simulink model "test_com_SensorFusion_SF_D4_ukf"  (R2019b)
settings: Solver=FixedStepDiscrete  StartTime=0  StopTime=stop  FixedStep=0.001  RelTol=1e-3
undefined symbols (not defined in the file or in its folder): breakpoints_camber_posZ, breakpoints_camber_RollAngle, BxTM, ByTM, camber_posZ_rear, camber_RollAngle_front, camber_RollAngle_rear, CxTM, CyTM, enable_kalman_standing, enable_simpleTireLoad_pGL, enable_v2o_direct, g, gamma_stat_front, gamma_stat_rear, gearbox_ratio, l_F, l_R, m_sprung, m_unsprung_quarter, mag_calib_front_center, mag_calib_front_compmatrix, mag_calib_rear_center, mag_calib_rear_compmatrix, should_be_in_theSensorFusion, switch_lat_accel_tireloadestimE8, switch_rocker_direction_FL, switch_rocker_direction_FR, switch_rocker_direction_RL, switch_rocker_direction_RR, switch_VelYcalculation_pSF, testStart_VelX_pSF, testVelY_pSF, tire_r_dyn, track_angle_front, track_width_front, track_width_rear, v2o_x, wheel_kinematics_breakpoints, wheel_kinematics_FL_data, wheel_kinematics_FR_data, wheelbase, x9DFrontX, x9DFrontY, x9DRearX, x9DRearY
libraries: SignalProcessingSensorFusionLib x30, simulink x9
(part 8 of 9)

== matlab function test_com_SensorFusion_SF_D4_ukf/Subsystem14/SensorFusion_D4/SF_LaKl_ukf ==
  data: x9DFront input Bus: control_9D; VehicleState output Bus: control_VehicleState; used_bias output Bus: control_bias_kalman_SiDe; used_measurements output Bus: control_used_measurements_SiDe; x9DRear input Bus: control_9D; v2o input Bus: control_Velocity; WheelSpeeds input; WheelSpeeds_Sq input; RockerAngle input; RockerAngle_Sq input; dt input; SteeringAngle input; bias_measurement_running output; kalman_running output; TireLoad output; TireSlipAngle output; TireSlipLong output; tire_r_dyn parameter; Rolling output; Pitching output; spring_stiff_roll_rear parameter; spring_stiff_heave_rear parameter; tire_cornering_stiffness parameter; wheel_inertia parameter; m_sprung parameter; m_unsprung_quarter parameter; damp_coef_heave_front_push parameter; damp_coef_heave_front_pull parameter; damp_coef_heave_rear_push parameter; damp_coef_roll_front_pull parameter; track_width_front parameter; track_width_rear parameter; spring_stiff_heave_front parameter; motion_ratio_heave_front parameter; motion_ratio_heave_rear parameter; wheelbase parameter; spring_stiff_roll_front parameter; motion_ratio_roll_front parameter; motion_ratio_roll_rear parameter; l_F parameter; l_R parameter; WheelTorque input; WheelAngle_FL input; WheelAngle_FR input; damp_coef_roll_front_push parameter; damp_coef_roll_rear_pull parameter; damp_coef_roll_rear_push parameter; damp_coef_heave_rear_pull parameter; Fx_tf_long input; Fy_tf_lat input; vehicle_inertia_yaw parameter; Fx_tf_long output; C_tl output; D_tl output; VelZ_eval output; PosZ output; TireLoad_z input; J_Sxx input; J_Syy input; x9DFrontX input; v2o_x input; chi output
function [VehicleState,used_bias,used_measurements,bias_measurement_running,kalman_running ,TireLoad, TireSlipAngle, TireSlipLong ,Rolling, Pitching, Fx_tf_long, C_tl,   D_tl, VelZ_eval, PosZ, chi]  = fcn(x9DFront, x9DRear, v2o, WheelSpeeds, WheelSpeeds_Sq, RockerAngle, RockerAngle_Sq, dt, SteeringAngle, tire_r_dyn,spring_stiff_roll_rear, spring_stiff_heave_rear, tire_cornering_stiffness, wheel_inertia, m_sprung, m_unsprung_quarter, damp_coef_heave_front_push, damp_coef_heave_front_pull, damp_coef_heave_rear_push, damp_coef_roll_front_pull, track_width_front, track_width_rear, spring_stiff_heave_front, motion_ratio_heave_front, motion_ratio_heave_rear, wheelbase, spring_stiff_roll_front, motion_ratio_roll_front, motion_ratio_roll_rear, l_F, l_R, WheelTorque, WheelAngle_FL, WheelAngle_FR, damp_coef_roll_front_push, damp_coef_roll_rear_pull, damp_coef_roll_rear_push, damp_coef_heave_rear_pull,Fx_tf_long, Fy_tf_lat, vehicle_inertia_yaw, TireLoad_z, J_Sxx, J_Syy, x9DFrontX, v2o_x)
%% SAE is the used KOS, global not local on the car -> trafo of measurements in global KOS necessary, but vel is local on the car?
persistent state P

persistent standstill_counter
persistent bias_measurements 
persistent P_bias

persistent YawAngle_Front_old YawAngle_Rear_old v2o_VelX_old RollAngle_Front_old PitchAngle_Front_old
persistent TireLoad_old chi_velocity velocity_old


num_states= 12;
num_measurements=7;


% state   =   (1) PosX
%             (2) PosY
%             (3) PosZ
%             (4) VelX
%             (5) VelY
%             (6) VelZ
%             (7) YawAngle
%             (8) RollAngle
%             (9) PitchAngle
%             (10) YawRate

     

% Actually used measurements:
%               (1) VelX
%               (2) VelY
%               (3) YawRate
%               (4) RollRate
%               (5) PitchRate



if isempty(P)
    
    P_bias=single(eye(num_measurements));%*0.01;
    standstill_counter=0;
    bias_measurements=single(zeros(num_measurements,1));
    

    state = single(zeros(num_states,1));
    P = single(eye(num_states, num_states)*10);
    
    YawAngle_Front_old=single(0);
    YawAngle_Rear_old=single(0);
    v2o_VelX_old=single(0);
    TireLoad_old= single([m_unsprung_quarter+0.5*m_sprung*l_R/wheelbase; ...
        m_unsprung_quarter + 0.5*m_sprung*l_R/wheelbase; ...
        m_unsprung_quarter + 0.5*m_sprung*l_F/wheelbase; ...
        m_unsprung_quarter + 0.5*m_sprung*l_F/wheelbase]);
    Fx_tf_long(1:4)=0;
    Fy_tf_lat(1:4)=0;
    chi_velocity = 0;
    velocity_old = [0;0];
end




%% Readability

PosX=       state(1);
PosY=       state(2);
PosZ=       state(3);
VelX=       state(4);
VelY=       state(5);
VelZ=       state(6);
RollAngle = state(7);
PitchAngle= state(8);
YawAngle=   state(9);
RollRate = state(10);
PitchRate = state(11);
YawRate =   state(12);

AccX_measurement = x9DFront.AccX;
AccY_measurement = x9DFront.AccY;
AccZ_measurement = x9DFront.AccZ;
YawRate_measurement = x9DFront.YawRate*1.167;%*0.8569;%; % the E9 Sensor had a wrong YawRate %*0.8569;%
RollRate_measurement = x9DFront.RollRate;
PitchRate_measurement = x9DFront.PitchRate;

chi = single(chi_velocity);

if isempty(YawAngle_Front_old)
    YawAngle_Front_old = single(0);
end
% 
if isempty(RollAngle_Front_old)
    RollAngle_Front_old = single(0);
end

if isempty(PitchAngle_Front_old)
    PitchAngle_Front_old = single(0);
end
YawAngle_measurement = single(0); %YawAngle_Front_old; %; 
RollAngle_measurement =  single(0);%RollAngle_Front_old; %
PitchAngle_measurement = single(0);% PitchAngle_Front_old;%
PosZ_measurement = single(0);
VelZ_measurement = single(0);

    measurements= [
        PosZ_measurement
v2o.VelX              % (1)  v2o Sensor  x velocity
v2o.VelY              % (2)  v2o Sensor  y velocity
VelZ_measurement
% RollAngle_measurement
% PitchAngle_measurement
RollRate_measurement
PitchRate_measurement
YawRate_measurement
];
% unused Pfusch-measurements (either integrating or giving zero dynamics)
% YawAngle_measurement
% RollAngle_measurement
% PitchAngle_measurement
% PosZ_measurement


measurements_Sq= [
    0
v2o.VelX_Sq            % (1)   v2o Sensor x velocity         Signal Quality
v2o.VelY_Sq            % (2)   v2o Sensor y velocity         Signal Quality
0
0
0
0];



%Correction of the sensor inputs with the estimated biases
% nb == no bias
measurements_nb=    measurements-bias_measurements;
PosZ_nb =           measurements_nb(1);
v2o_VelX_nb=        measurements_nb(2);
v2o_VelY_nb=        measurements_nb(3);
VelZ_nb=            measurements_nb(4);
% AccX_nb =           measurements_nb(5);
% AccY_nb =           measurements_nb(6);
% AccZ_nb =           measurements_nb(7);
% RollAngle_nb =      measurements_nb(8);
% PitchAngle_nb =     measurements_nb(9);
%YawAngle_nb =       measurements_nb(10);
RollRate_nb =       measurements_nb(5);
PitchRate_nb =      measurements_nb(6);
YawRate_nb =        measurements_nb(7);                

Q=diag([0.00001   %(1) PosX 01E-8
        0.0001   %(2) PosY 01E-8
        0.001    %(3) PosZ 1E-6
        0.001    %(4) VelX 0.001
        0.001     %(5) VelY 0.001
        1    %(6) VelZ 0,1 
        0.0001    %(10) RollAngle 0.001
        0.0001   % (11)  PitchAngle 0.0001
        0.00001    %(12) YawAngle 0.001
        0.00001    %(13)RollRate
        0.00001      %(14) PitchRate
        0.00001]);   %(15) YawRate 

%Measurement noise Covariance matrix
    
R=diag([0.01  %(1) PosZ
        0.01   % (1) VelX 1E-3
        0.01   % (2) VelY 1E-3
        1    % (3) VelZ 
        0.001    % (7) RollRate
        0.001   % (8) PitchRate
        0.001 ]);   % (7) YawRate
%         0.001    % (8) PitchRate 
%         0.0001 % (9) YawRate 
%         
     
avgWheelSpeed=mean(abs(WheelSpeeds));


if (avgWheelSpeed < 0.02 )
        vehicle_is_driving=false;
        standstill_counter=standstill_counter+1;
else
        vehicle_is_driving=true;
        standstill_counter=0;
end

bias_measurement_running=false;
kalman_running=false;

%vehicle_is_driving = true;

RollAngle = state(8);
PitchAngle = state(9);

%Verwendete Messung für v2o VelX
use_v2o_VelX=0;
v2o_VelX_used_measurement=single(0);
if (v2o.VelX_Sq<4) && (v2o.VelY_Sq<4) && abs(v2o_VelX_nb-v2o_VelX_old) < 2
    
    v2o_VelX_used_measurement=v2o_VelX_nb;

    use_v2o_VelX=1;

end

if(v2o_VelX_old~=v2o_VelX_nb)
    v2o_VelX_old=v2o_VelX_nb;
end

% 0.221 = r_dyn vom Reifen : v = r*omega
% Chi square test to validate velocity measurement and estimation
if chi_velocity>4
    v2o_VelX_nb = single((WheelSpeeds(3)+WheelSpeeds(4)+cosd(SteeringAngle)*(WheelSpeeds(1)+WheelSpeeds(2)))*0.221/(4));
    v2o_VelY_nb = single(sind(SteeringAngle)*(WheelSpeeds(1)+WheelSpeeds(2))*0.221);
end


% measurement vector
zmeas  = [PosZ_nb;...
    v2o_VelX_nb;...
    v2o_VelY_nb;...
    VelZ_nb;...
    RollRate_nb;...
    PitchRate_nb;...
    YawRate_nb];

% calculate TF_Fx_front and TF_Fy_rear and TF_Fy_front

TF_Fx_F = Fx_tf_long(1)+Fx_tf_long(2);
TF_Fy_F = Fy_tf_lat(1)+Fy_tf_lat(2);
TF_Fy_R = Fy_tf_lat(3)+Fy_tf_lat(4);
TF_Fx_R = Fx_tf_long(3)+Fx_tf_long(4);

u = [WheelSpeeds(1);... % FL
    WheelSpeeds(2);...  % FR
    WheelSpeeds(3);...  % RL
    WheelSpeeds(4);...  % RR
    AccX_measurement;...
    AccY_measurement;...
    AccZ_measurement;...
    vehicle_inertia_yaw;...
    J_Sxx;...
    J_Syy;...
    TF_Fx_F;...
    TF_Fx_R;...
    TF_Fy_F;...
    TF_Fy_R;...
    TireLoad_z(1);...
    TireLoad_z(2);...
    TireLoad_z(3);...
    TireLoad_z(4);...
    SteeringAngle;...
    l_F;...
    l_R;...
    wheelbase;...
    track_width_front;...
    track_width_rear];

u_param = [x9DFrontX
    v2o_x];


%% Kalman-Filtering START
if (~vehicle_is_driving)
    

    if standstill_counter*dt>2 && standstill_counter*dt<10
    bias_measurement_running=true;    
    kill_matrix_bias=zeros(num_measurements,num_measurements);
        for i=1:num_measurements
            if measurements_Sq(i)<4
                kill_matrix_bias(i,i)=1;
            end
        end
        H_bias=kill_matrix_bias;
        R_bias=eye(num_measurements)*0.01;  % Sinnvolle Werte?
        I_bias=eye(num_measurements);
        
        Z_bias = kill_matrix_bias*measurements;
        w_bias = Z_bias-(H_bias*bias_measurements);
        K_bias = (P_bias*H_bias')/(H_bias*P_bias*H_bias.'+R_bias);  
        bias_measurements = bias_measurements+K_bias*w_bias;
        P_bias = (I_bias-K_bias*H_bias)*P_bias;
    end

    
    
    
    
else 
        
    kalman_running=true;
    fstate = @(x)f(x,u,dt);
    hmeas =@(x)h(x, u_param);



    % Unscented Kalman Filtering 
    [state,P,S,r1,r2]=ukf(fstate,state,P,hmeas,zmeas,Q,R);

    % try chi-square test for velocity
    r = r2(2:3)-r1(2:3);
    chi = r'*inv(S(2:3,2:3))*r;

    % if chi > bestimmter value -> von V2O auf Wheelspeeds als Signal umsteigen
    chi_velocity = double(chi);
end


% Plausibility check
if VelX<0
    VelX=single(0);
end

if ~vehicle_is_driving
    VelX=single(0); 
    VelY=single(0); 
    YawRate=single(0); 
end




VehicleState.PosX = PosX; % state(1);
VehicleState.PosY = PosY; % state(2);
VehicleState.VelX = VelX; % state(4);
VehicleState.VelY = VelY; % state(5);
VehicleState.YawAngle = YawAngle; % state(9);
VehicleState.YawRate = YawRate; % state(12);
VehicleState.YawAcc = single(0);
VehicleState.AccX = AccX_measurement;
VehicleState.AccY = AccY_measurement;
VehicleState.AccZ = AccZ_measurement;
VehicleState.isDriving = vehicle_is_driving;

Rolling = RollAngle;% state(7);
Pitching = PitchAngle; % state(8);
YawRate = YawRate; % state(12);

used_bias.VelX_bias=bias_measurements(1);
used_bias.VelY_bias=bias_measurements(2);
used_bias.YawAngle_9DFront_bias= single(0); %bias_measurements(3);
used_bias.YawRate_9DFront_bias=single(0); %bias_measurements(4);
used_bias.YawAngle_9DRear_bias=single(0);
used_bias.YawRate_9DRear_bias=single(0);
used_bias.wheelvelocity_FL_bias=single(0); %bias_measurements(5);
used_bias.wheelvelocity_FR_bias=single(0); %bias_measurements(6);
used_bias.wheelvelocity_RL_bias=single(0); %bias_measurements(7);
used_bias.wheelvelocity_RR_bias=single(0); %bias_measurements(8);


used_measurements.VelX_measurement=zmeas(1);
used_measurements.VelY_measurement=zmeas(2);
used_measurements.YawAngle_9DFront_measurement = single(0); %z(3);


used_measurements.YawRate_9DFront_measurement=zmeas(7); %z(4);
used_measurements.YawAngle_9DRear_measurement=single(0);
used_measurements.YawRate_9DRear_measurement=single(0);
used_measurements.wheelvelocity_FL_measurement=single(0); %z(5);
used_measurements.wheelvelocity_FR_measurement=single(0); %z(6);
used_measurements.wheelvelocity_RL_measurement=single(0); %z(7);
used_measurements.wheelvelocity_RR_measurement=single(0); %z(8);
YawAngle_Front_old = state(12);
RollAngle_Front_old = state(10);
PitchAngle_Front_old = state(11);
VelZ_eval = state(6);

%% Tire Load Estimation to improve Yaw Angle Estimation

% formula: tl= C_tl+D_tl;

% MonoShock Auswahl Druck/Zug-Stufe
if -PitchRate*l_F + PosZ > 0  %Vorne Druck
    damp_coef_heave_front = damp_coef_heave_front_push;
else                    %Vorne Zug
    damp_coef_heave_front = damp_coef_heave_front_pull;
end

if PitchRate*l_R + PosZ > 0  %Hinten Druck
    damp_coef_heave_rear = damp_coef_heave_rear_push;
else                    %Hinten Zug
    damp_coef_heave_rear = damp_coef_heave_rear_pull;
end


% Rolldämpfer Auswahl Druck/Zug-Stufe
if RollRate < 0 
    % if Bedingung muss überprüft werden!
    damp_coef_roll_front = damp_coef_roll_front_push;
    damp_coef_roll_rear = damp_coef_roll_rear_push;
else
    damp_coef_roll_front = damp_coef_roll_front_pull;
    damp_coef_roll_rear = damp_coef_roll_rear_pull; 
end
damp_F=@(v,damp_coef)(v*0.5*(damp_coef(2)+damp_coef(3))+sign(v)*(0.5*(damp_coef(2)-damp_coef(3))*(damp_coef(1)-abs(v*sign(v)-damp_coef(1)))));

%Nicht-Lineare Ausgangsmatrix
C_tl = [  (2*motion_ratio_heave_front^2*spring_stiff_heave_front*PosZ+ motion_ratio_heave_front*damp_F(2*motion_ratio_heave_front*VelZ,damp_coef_heave_front)  -track_width_front*motion_ratio_roll_front^2*spring_stiff_roll_front*RollAngle+  motion_ratio_roll_front*damp_F(-track_width_front*motion_ratio_roll_front*RollRate,damp_coef_roll_front)  -2*l_F*motion_ratio_heave_front^2*spring_stiff_heave_front*PitchAngle+  motion_ratio_heave_front*damp_F(-2*l_F*motion_ratio_heave_front*PitchRate,damp_coef_heave_front));
          (2*motion_ratio_heave_front^2*spring_stiff_heave_front*PosZ+ motion_ratio_heave_front*damp_F(2*motion_ratio_heave_front*VelZ,damp_coef_heave_front)+  track_width_front*motion_ratio_roll_front^2*spring_stiff_roll_front*RollAngle+   motion_ratio_roll_front*damp_F(track_width_front*motion_ratio_roll_front*RollRate,damp_coef_roll_front)  -2*l_F*motion_ratio_heave_front^2*spring_stiff_heave_front*PitchAngle+  motion_ratio_heave_front*damp_F(-2*l_F*motion_ratio_heave_front*PitchRate,damp_coef_heave_front));
            (2*motion_ratio_heave_rear^2*spring_stiff_heave_rear*PosZ+    motion_ratio_heave_rear*damp_F(2*motion_ratio_heave_rear*VelZ,damp_coef_heave_rear)     -track_width_rear*motion_ratio_roll_rear^2*spring_stiff_roll_rear*RollAngle+      motion_ratio_roll_rear*damp_F(-track_width_rear*motion_ratio_roll_rear*RollRate,damp_coef_roll_rear)+    2*l_R*motion_ratio_heave_rear^2*spring_stiff_heave_rear*PitchAngle+      motion_ratio_heave_rear*damp_F(2*l_R*motion_ratio_heave_rear*PitchRate,damp_coef_heave_rear));
            (2*motion_ratio_heave_rear^2*spring_stiff_heave_rear*PosZ+    motion_ratio_heave_rear*damp_F(2*motion_ratio_heave_rear*VelZ,damp_coef_heave_rear)+     track_width_rear*motion_ratio_roll_rear^2*spring_stiff_roll_rear*RollAngle+       motion_ratio_roll_rear*damp_F(track_width_rear*motion_ratio_roll_rear*RollRate,damp_coef_roll_rear)+    2*l_R*motion_ratio_heave_rear^2*spring_stiff_heave_rear*PitchAngle+      motion_ratio_heave_rear*damp_F(2*l_R*motion_ratio_heave_rear*PitchRate,damp_coef_heave_rear))];
g=9.81;
        
D_tl = [m_unsprung_quarter + 0.5*m_sprung*l_R/wheelbase; 
        m_unsprung_quarter + 0.5*m_sprung*l_R/wheelbase; 
        m_unsprung_quarter + 0.5*m_sprung*l_F/wheelbase; 
        m_unsprung_quarter + 0.5*m_sprung*l_F/wheelbase]*g;

TireLoad = C_tl  + D_tl;

%Begrenzung der Radlast
for n=1:1:4
    if TireLoad(n) > 1800
        TireLoad(n) = 1800;
    elseif TireLoad(n) < 0
        TireLoad(n) = 0;
    end
end

TireLoad_old = TireLoad;

%% Berechnung des TireSlipAngle und TireSlipLongitudinal

%%Friction Estimation
vel = ([VelX; VelY; 0]);  
acc = ([AccX_measurement;AccY_measurement;0]);
Rad = [l_F, l_F, -l_R, -l_R; -track_width_front/2, track_width_front/2, -track_width_rear/2, track_width_rear/2; 0, 0, 0, 0];  %Abstand cog zu rad mitte


% v_r = omega*r - v_x
% wheelAngleLeft/Right: positiv bei Rechtskurve
% gierrate positiv bei rechtskurve

% define velocity vector for CoG
% vel(1) = x(1);
% vel(2) = x(2) - x(14)*v2o_x; % checken ob evtl Vorzeichen vertauscht werden muss
% vel(3) = 0;%TODO:wenn gefilterte, plausible Werte von Sensorfusion, dann hier dazunehmen

% define acceleration vector for CoG
% acc(1) = x(5);
% acc(2) = x(6);
% acc(3) = 0;%TODO:wenn gefilterte, plausible Werte von Sensorfusion, dann hier dazunehmen

% define yaw rate and yaw acceleration of CoG
% yawRate = x(15);
% yawAcc = x(16); 

%% Rösselsprung-Matrizen für Rotation
omegaTilde = [0,-YawRate,PitchRate;  
                YawRate,0,-RollRate;
                    -PitchRate,RollRate,0];
% omegaDotTilde = [0,-YawAcc,PitchAcc;
%                    YawAcc,0,-RollAcc;
%                     -PitchAcc,RollAcc,0];
%        
% omegaTilde = [0,-YawRate,0;...  % hier eigentlich noch Pitch und roll rate
%                 YawRate,0,0;...
%                     0,0,0];
% omegaDotTilde = [0,-YawAcc,0;...
%                    YawAcc,0,0;...
%                     0,0,0];                

% velocity of tires 
velTire_FL = vel + omegaTilde * Rad(:,1);
velTire_FR = vel + omegaTilde * Rad(:,2);
velTire_RL = vel + omegaTilde * Rad(:,3);
velTire_RR = vel + omegaTilde * Rad(:,4);

velTire = [velTire_FL; velTire_FR; velTire_RL; velTire_RR];
% acceleration of tires %TODO: Passende Formel aus
% Maschinendynamik raussuchen und verifizieren
% accTire_FL = acc + omegaDotTilde * Rad(:,1) + omegaTilde * (omegaTilde * Rad(:,1)); 
% accTire_FR = acc + omegaDotTilde * Rad(:,2) + omegaTilde * (omegaTilde * Rad(:,2));
% accTire_RL = acc + omegaDotTilde * Rad(:,3) + omegaTilde * (omegaTilde * Rad(:,3));
% accTire_RR = acc + omegaDotTilde * Rad(:,4) + omegaTilde * (omegaTilde * Rad(:,4));
% 
% accTire= [accTire_FL; accTire_FR; accTire_RL; accTire_RR];

%% Rotational matrices for Transformation from car coordinate system 
% into wheel coordinate systems
% rotMatrix_Front = [cos(delta),sin(delta),0; ... % hier eigentlich auch noch roll und pitch angle
%               -sin(delta),cos(delta),0;...
%               0,0,1];

rotMatrix_FL = [cos(WheelAngle_FL),sin(WheelAngle_FL),0; ... % hier eigentlich auch noch roll und pitch angle
              -sin(WheelAngle_FL),cos(WheelAngle_FL),0;...
              0,0,1];
          
rotMatrix_FR = [cos(WheelAngle_FR),sin(WheelAngle_FR),0; ... % hier eigentlich auch noch roll und pitch angle
              -sin(WheelAngle_FR),cos(WheelAngle_FR),0;...
              0,0,1];
rotMatrix_Rear = [1,0,0; 0,1,0; 0,0,1];
          
          
%% Transformationsmatrixen von Vehicle cog zu den einzelnen Rädern mit Roll und Pitchangle
% inverse von (11.9 und 11.10) für vorne und hinten
% rotMatrix_Front=[cos(delta)*cos(PitchAngle),-sin(delta)*cos(PitchAngle),-sin(PitchAngle);  % hier eigentlich auch noch roll und pitch angle
%               sin(RollAngle)*sin(PitchAngle)*cos(delta)-sin(delta)*cos(RollAngle),...
%               -sin(RollAngle)*sin(PitchAngle)*sin(WheelAngle(1)+cos(WheelAngle(1))*cos(RollAngle),...
%               sin(RollAngle)*cos(PitchAngle));
%               cos(RollAngle)*sin(PitchAngle)*cos(delta)-sin(RollAngle)*sin(delta),...
%                   -cos(RollAngle)*sin(PitchAngle)*sin(delta)-sin(RollAngle)*cos(delta),cos(RollAngle)*cos(PitchAngle)];
% 
% rotMatrix_Rear=([cos(PitchAngle),0, -sin(PitchAngle); 
%               sin(RollAngle)*sin(PitchAngle),cos(RollAngle),sin(RollAngle)*cos(PitchAngle);
%               cos(RollAngle)*sin(PitchAngle),-sin(RollAngle), cos(RollAngle)*cos(PitchAngle)]);

% velocity of tires in tire coordinats (dieses Superpositionsprinzip ändert sich bei beta
% ungleich 0)
% wenn andere transformationsmatrix * durhch \ ersetzen
vel_help_FL = rotMatrix_FL * velTire_FL;
velX_FL = vel_help_FL(1);
velY_FL = vel_help_FL(2);
vel_help_FR = rotMatrix_FR* velTire_FR;
velX_FR = vel_help_FR(1);
velY_FR = vel_help_FR(2);
vel_help_RL = rotMatrix_Rear*velTire_RL;
velX_RL = vel_help_RL(1);
velY_RL = vel_help_RL(2);
vel_help_RR = rotMatrix_Rear*velTire_RR;
velX_RR = vel_help_RR(1);
velY_RR = vel_help_RR(2);

velX= single([velX_FL, velX_FR, velX_RL, velX_RR]);
velY= single([velY_FL, velY_FR, velY_RL, velY_RR]);

% % acceleration of tires in tire coordinates
% acc_FL = rotMatrix_FL * accTire_FL;
% accX_FL = acc_FL(1);
% acc_FR = rotMatrix_FR* accTire_FR;
% accX_FR = acc_FR(1);
% acc_RL = rotMatrix_Rear* accTire_RL;
% accX_RL = acc_RL(1);
% acc_RR = rotMatrix_Rear*accTire_RR;
% accX_RR = acc_RR(1);
% accX=[accX_FL, accX_FR, accX_RL, accX_RR];

WheelVelocity_FL = WheelSpeeds(1);
WheelVelocity_FR = WheelSpeeds(2);
WheelVelocity_RL = WheelSpeeds(3);
WheelVelocity_RR = WheelSpeeds(4);

% relative velocities of wheels
velRelX_FL = WheelVelocity_FL - velX_FL;  %hier später die Zustände aus dem kalman filter für wheelspeeds
velRelX_FR = WheelVelocity_FR - velX_FR;
velRelX_RL = WheelVelocity_RL - velX_RL;
velRelX_RR = WheelVelocity_RR - velX_RR;

velRelX= [velRelX_FL; velRelX_FR; velRelX_RL; velRelX_RR];

if(velX*ones(4,1) < 0.4) %TODO: Nachschauen, ob die Schwelle Probleme bereitet, oder ob diese höher oder tiefer gesetzt werden muss
    TireSlipLong = single([0, 0, 0, 0].');
else    		
TireSlipLong = [(velRelX_FL/max(abs(velX_FL), abs(WheelVelocity_FL))); (velRelX_FR/max(abs(velX_FR), abs(WheelVelocity_FR)));...
        (velRelX_RL/max(abs(velX_RL), abs(WheelVelocity_RL)));(velRelX_RR/max(abs(velX_RR), abs(WheelVelocity_RR)))];
end   


if(velX*ones(4,1) < 0.4)
    TireSlipAngle = single([0, 0, 0, 0].');
else
     TireSlipAngle = [-atan(velY_FL)/(abs(velX_FL)); ...
        -atan(velY_FR)/(abs(velX_FR));... % hier müssen dann die Zustände von kalman mit mal r übertragen werden
        -atan(velY_RL)/(abs(velX_RL));...
       -atan(velY_RR)/(abs(velX_RR))];   
end

for n=1:1:4
    if TireSlipLong(n) > 1
        TireSlipLong(n) = 1;
    elseif TireSlipLong(n) < -1
        TireSlipLong(n) = -1;
    end
end
%mit v=omega*r und alpha=omega/t=omega*r/(t*r)=a/r
% WheelSpeedNoSlip = velX.'/(tire_r_dyn);
%WheelAccNoSlip = accX.'/(tire_r_dyn);

end

function [x,P,P2,z,z1]=ukf(fstate,x,P,hmeas,z,Q,R)
% UKF   Unscented Kalman Filter for nonlinear dynamic systems
% [x, P] = ukf(f,x,P,h,z,Q,R) returns state estimate, x and state covariance, P 
% for nonlinear dynamic system (for simplicity, noises are assumed as additive):
%           x_k+1 = f(x_k) + w_k
%           z_k   = h(x_k) + v_k
% where w ~ N(0,Q) meaning w is gaussian noise with covariance Q
%       v ~ N(0,R) meaning v is gaussian noise with covariance R
% Inputs:   f: function handle for f(x)
%           x: "a priori" state estimate
%           P: "a priori" estimated state covariance
%           h: fanction handle for h(x)
%           z: current measurement
%           Q: process noise covariance 
%           R: measurement noise covariance
% Output:   x: "a posteriori" state estimate
%           P: "a posteriori" state covariance
%
% Example:
%{
n=3;      %number of state
q=0.1;    %std of process 
r=0.1;    %std of measurement
Q=q^2*eye(n); % covariance of process
R=r^2;        % covariance of measurement  
f=@(x)[x(2);x(3);0.05*x(1)*(x(2)+x(3))];  % nonlinear state equations
h=@(x)x(1);                               % measurement equation
s=[0;0;1];                                % initial state
x=s+q*randn(3,1); %initial state          % initial state with noise
P = eye(n);                               % initial state covraiance
N=20;                                     % total dynamic steps
xV = zeros(n,N);          %estmate        % allocate memory
sV = zeros(n,N);          %actual
zV = zeros(1,N);
for k=1:N
  z = h(s) + r*randn;                     % measurments
  sV(:,k)= s;                             % save actual state
  zV(k)  = z;                             % save measurment
  [x, P] = ukf(f,x,P,h,z,Q,R);            % ekf 
  xV(:,k) = x;                            % save estimate
  s = f(s) + q*randn(3,1);                % update process 
end
for k=1:3                                 % plot results
  subplot(3,1,k)
  plot(1:N, sV(k,:), '-', 1:N, xV(k,:), '--')
end
%}
% Reference: Julier, SJ. and Uhlmann, J.K., Unscented Filtering and
% Nonlinear Estimation, Proceedings of the IEEE, Vol. 92, No. 3,
% pp.401-422, 2004. 
%
% By Yi Cao at Cranfield University, 04/01/2008
%
L=numel(x);                                 %numer of states
m=numel(z);                                 %numer of measurements
alpha=1e-3;                                 %default, tunable
ki=0;                                       %default, tunable
beta=2;                                     %default, tunable
lambda=alpha^2*(L+ki)-L;                    %scaling factor
c=L+lambda;                                 %scaling factor
Wm=[lambda/c 0.5/c+zeros(1,2*L)];           %weights for means
Wc=Wm;
Wc(1)=Wc(1)+(1-alpha^2+beta);               %weights for covariance
c=sqrt(c);
X=sigmas(x,P,c);                            %sigma points around x
[x1,X1,P1,X2]=ut(fstate,X,Wm,Wc,L,Q);          %unscented transformation of process
% X1=sigmas(x1,P1,c);                         %sigma points around x1
% X2=X1-x1(:,ones(1,size(X1,2)));             %deviation of X1
[z1,Z1,P2,Z2]=ut(hmeas,X1,Wm,Wc,m,R);       %unscented transformation of measurments
P12=X2*diag(Wc)*Z2';                        %transformed cross-covariance
K=P12*inv(P2);
x=x1+K*(z-z1);                              %state update
P_=P1-K*P12';                                %covariance update
P=single(P_);
end

function [y,Y,P,Y1]=ut(f,X,Wm,Wc,n,R)
%Unscented Transformation
%Input:
%        f: nonlinear map
%        X: sigma points
%       Wm: weights for mean
%       Wc: weights for covraiance
%        n: numer of outputs of f
%        R: additive covariance
%Output:
%        y: transformed mean
%        Y: transformed smapling points
%        P: transformed covariance
%       Y1: transformed deviations

L=size(X,2);
y=zeros(n,1);
Y=zeros(n,L);
for k=1:L                   
    Y(:,k)=f(X(:,k));       
    y=y+Wm(k)*Y(:,k);       
end
Y1=Y-y(:,ones(1,L));
P=Y1*diag(Wc)*Y1'+R;          
end

function X=sigmas(x,P,c)
%Sigma points around reference point
%Inputs:
%       x: reference point
%       P: covariance
%       c: coefficient
%Output:
%       X: Sigma points

A = c*chol(P)';
Y = x(:,ones(1,numel(x)));
X = [x Y+A Y-A]; 
end

function x_dot=f(x,u,dt)
% Systemgleichung x_dot = f(x)
% 
% Zustandsvektor x
PosX = x(1);
PosY = x(2);
PosZ = x(3);
VelX = x(4);
VelY = x(5);
VelZ = x(6);
RollAngle = x(7);
PitchAngle = x(8);
YawAngle = x(9);
RollRate = x(10);
PitchRate = x(11);
YawRate = x(12);

% Eingangssignal u
WheelSpeeds_FL = u(1);% FL
WheelSpeeds_FR = u(2); % FR
WheelSpeeds_RL = u(3); % RL
WheelSpeeds_RR = u(4); % RR
AccX = u(5);
AccY = u(6);
AccZ = u(7);
J_zz = u(8);
J_xx = u(9);
J_yy = u(10);
TF_Fx_F = u(11);
TF_Fx_R = u(12);
TF_Fy_F = u(13);
TF_Fy_R = u(14);
TF_Z_FL = u(15);
TF_Z_FR = u(16);
TF_Z_RL = u(17);
TF_Z_RR = u(18);
SteeringAngle = u(19);
l_F = u(20);
l_R = u(21);
wheelbase = u(22); % -> not needed
track_width_front = u(23);
track_width_rear = u(24);


WheelSpeed_max = max(u(1:4));

if WheelSpeed_max<0.5
    YawRate_WS = 0;
else
    YawRate_WS_Front = (WheelSpeeds_FR-WheelSpeeds_FL)*0.221/(track_width_front*cosd(SteeringAngle));
    YawRate_WS_Rear = (WheelSpeeds_RR-WheelSpeeds_RL)*0.221/(track_width_rear);
    YawRate_WS = double(0.5*(YawRate_WS_Front+YawRate_WS_Rear));
end

%implementing it not discrete but continous
x_dot=[PosX+VelX*dt %PosX+cos(YawAngle)*dt*VelX+sin(YawAngle)*VelY*dt  %(cosd(SteeringAngle)*(WheelSpeeds_FL+WheelSpeeds_FR)+WheelSpeeds_RL+WheelSpeeds_RR)/4*dt+PosX% 
    PosY + VelY*dt  %PosY-sin(YawAngle)*VelX*dt+dt*VelY*cos(YawAngle)  %sind(SteeringAngle)*(WheelSpeeds_FR+WheelSpeeds_FL)/2*dt+PosY  %
    VelZ*dt+PosZ
    (AccX+VelY*YawRate)*dt+VelX
    (AccY-VelX*YawRate)*dt+VelY
    AccZ*dt+VelZ
    RollAngle+RollRate*dt
    PitchAngle+dt*PitchRate
    YawAngle+dt*YawRate_WS
    RollRate   %(track_width_front/2*(TF_Z_FL+TF_Z_FR-TF_Z_RL-TF_Z_RR))/J_xx*dt+RollRate % 
    PitchRate  %(l_F*(TF_Z_FL+TF_Z_FR)-l_R*(TF_Z_RL+TF_Z_RR))/J_yy*dt+PitchRate  %
    YawRate_WS];  %YawRate]; %];(track_width_front/2*(cos(SteeringAngle)*TF_Fx_F+sin(SteeringAngle)*TF_Fy_F-(-sin(SteeringAngle)*TF_Fx_F+cos(SteeringAngle)*TF_Fy_F)+TF_Fx_R)+l_F*(TF_Fy_F)-l_R*(TF_Fy_R))/J_zz*dt+YawRate



% PosX+cos(YawAngle)*dt*VelX+sin(YawAngle)*VelY*dt;  %(1) PosX
%              PosY-sin(YawAngle)*VelX*dt+dt*VelY*cos(YawAngle);  %(2) PosY
%              PosZ+VelZ*dt;                       %(3) PosZ
%              VelX+dt*(AccX+VelY*YawRate);               %%%%VelX+cos(YawAngle)*AccX*dt-sin(YawAngle)*YawRate*VelX*dt+sin(YawAngle)*AccY+cos(YawAngle)*YawRate*VelY*dt                       %(4) VelX
%              VelY+dt*(AccY-VelX*YawRate);               %%%%%VelY-sin(YawAngle)*AccX*dt-cos(YawAngle)*YawRate*VelX*dt+cos(YawAngle)*AccY-sin(YawAngle)*YawRate*VelY*dt                     %(5) VelY
%              VelZ+AccZ*dt;              %(6) VelZ
%              AccX_sig;
%              AccY_sig;
%              AccZ_sig + 9.81;
%              RollAngle+dt*RollRate;
%              PitchAngle+dt*PitchRate;
%              YawAngle+dt*YawRate;
%              RollRate_sig;
%              PitchRate_sig;
%              YawRate_sig];
%             %((TF_Fx_F*cos(SteeringAngle)+TF_Fy_F*sin(SteeringAngle))*l_F-TF_Fy_R*l_R)/Inertia_Yaw ];
% 
%             
            
end

function z=h(x, u_param)
% Messgleichung y = h(x)
x9d_F_x = u_param(1);
v2o_x= u_param(2);

z=[x(3);...
    v2o_x+x(4);...
    v2o_x+x(5);...
    x(6);...
    x9d_F_x+x(10);...
    x9d_F_x+x(11);... % Berücksichtigung von Corioliskräften?
    x9d_F_x+x(12)];
    
end

== matlab function test_com_SensorFusion_SF_D4_ukf/Subsystem14/SensorFusion_D4/MATLAB Function ==
  data: DriverDemand input; VehicleState output Bus: control_VehicleState; WheelSpeeds input; WheelAngle input; tire_r_dyn parameter; dt input single; l_F parameter; l_R parameter; TireSlipLong output; WheelVelocity output; WheelVelocity_old input single size=4; track_width_front parameter; track_width_rear parameter; wheelbase parameter
function [VehicleState, TireSlipLong, WheelVelocity] = Sensorless(DriverDemand, WheelSpeeds, WheelAngle, tire_r_dyn, dt, l_F, l_R, WheelVelocity_old, track_width_front, track_width_rear, wheelbase) 

% diese Funktion ist dafür da, wenn mit keinen Sensoren gefahren wird
% (Anfang der Saison)

WheelVelocity=tire_r_dyn*WheelSpeeds;
WheelVelocity_FL=WheelVelocity(1);
WheelVelocity_FR=WheelVelocity(2);
WheelVelocity_RL=WheelVelocity(3);
WheelVelocity_RR=WheelVelocity(4);

VelX_FL=(WheelVelocity(1))*cos(WheelAngle(1));
VelX_FR=WheelVelocity(2)*cos(WheelAngle(2)); %beim Beschleunigen HInterradantrieb, die Vorderen Räder sind stabiler, kein Schlupf
    
VelX=(VelX_FL+VelX_FR+WheelVelocity_RL+WheelVelocity_RR)/4;
AccX=single(0); 
TireSlipLong=[single(0); single(0); single(0); single(0)];

    WheelAcc_FL=(WheelVelocity_FL-WheelVelocity_old(1))/dt;
    WheelAcc_FR=(WheelVelocity_FR-WheelVelocity_old(2))/dt;
if DriverDemand>=0 
    VelX=(VelX_FL+VelX_FR)*0.5;
    AccX=(WheelAcc_FL+WheelAcc_FR)*0.5; 
    TireSlipLong=[single(0); single(0); -(WheelVelocity_RL-VelX)/max(abs(VelX), abs(WheelVelocity_RL)); -(WheelVelocity_RR-VelX)/max(abs(VelX), abs(WheelVelocity_RR))]; 
end    
   VelX_RL=(WheelVelocity(3));
    VelX_RR=WheelVelocity(4);
    WheelAcc_RL=(WheelVelocity_RL-WheelVelocity_old(3))/dt;
    WheelAcc_RR=(WheelVelocity_RR-WheelVelocity_old(4))/dt;   
if DriverDemand<0 % im Bremsfall, nur Vorderräder gebremst
    VelX=(VelX_RL+VelX_RR)*0.5;
    AccX=(WheelAcc_RL+WheelAcc_RR)*0.5;
    TireSlipLong=[(-(WheelVelocity_FL-VelX*cos(WheelAngle(1)))/max(abs(VelX*cos(WheelAngle(1))), abs(WheelVelocity_FL))); -((WheelVelocity_FR-VelX*cos(WheelAngle(2)))/max(abs(VelX*cos(WheelAngle(2))), abs(WheelVelocity_FR))); single(0); single(0)]; 
end  

%vel=YawRate*R einspurmodell

delta=(WheelAngle(1)+WheelAngle(2))*0.5;
r_y=single((wheelbase-VelX*0.03+0.0)*tan(sign(delta)*(pi*0.5)-0.2047*3.76*delta));

YawRate=(VelX*delta)/(l_F+l_R);
AccY=VelX*YawRate;
%VelY=(AccY-AccY_old)*dt;
%YawAcc=(YawRate-YawRate_old)/dt;



PosX=single(0);
PosY=single(0);
AccZ=single(0);
YawAngle=single(0);
YawAcc=single(0);
VelY=single(0);

VehicleState.PosX = PosX;
VehicleState.PosY = PosY;
VehicleState.VelX = VelX;
VehicleState.VelY = VelY;
VehicleState.YawAngle = YawAngle;
VehicleState.YawRate = YawRate;
VehicleState.YawAcc = YawAcc;
VehicleState.AccX = AccX;
VehicleState.AccY = AccY;
VehicleState.AccZ = AccZ;
VehicleState.isDriving = true;

vel = ([VelX; VelY; 0]);  
Rad = [l_F, l_F, -l_R, -l_R; -track_width_front/2, track_width_front/2, -track_width_rear/2, track_width_rear/2; 0, 0, 0, 0];  %Abstand cog zu rad mitte

       
omegaTilde = [0,-YawRate,0;...  % hier eigentlich noch Pitch und roll rate
                YawRate,0,0;...
                    0,0,0];

% velocity of tires 
velTire_FL = vel + omegaTilde * Rad(:,1);
velTire_FR = vel + omegaTilde * Rad(:,2);
velTire_RL = vel + omegaTilde * Rad(:,3);
velTire_RR = vel + omegaTilde * Rad(:,4);


%% Rotational matrices for Transformation from car coordinate system 
% into wheel coordinate systems
% rotMatrix_Front = [cos(delta),sin(delta),0; ... % hier eigentlich auch noch roll und pitch angle
%               -sin(delta),cos(delta),0;...
%               0,0,1];
WheelAngle_FL=WheelAngle(1);
WheelAngle_FR=WheelAngle(2);          
rotMatrix_FL = [cos(WheelAngle_FL),sin(WheelAngle_FL),0; ... % hier eigentlich auch noch roll und pitch angle
              -sin(WheelAngle_FL),cos(WheelAngle_FL),0;...
              0,0,1];
          
rotMatrix_FR = [cos(WheelAngle_FR),sin(WheelAngle_FR),0; ... % hier eigentlich auch noch roll und pitch angle
              -sin(WheelAngle_FR),cos(WheelAngle_FR),0;...
              0,0,1];
rotMatrix_Rear = [1,0,0; 0,1,0; 0,0,1];
 

% velocity of tires in tire coordinats (dieses Superpositionsprinzip ändert sich bei beta
% ungleich 0)
% wenn andere transformationsmatrix * durhch \ ersetzen
vel_help_FL = rotMatrix_FL * velTire_FL;
velX_FL = vel_help_FL(1);
velY_FL = vel_help_FL(2);
vel_help_FR = rotMatrix_FR* velTire_FR;
velX_FR = vel_help_FR(1);
velY_FR = vel_help_FR(2);
vel_help_RL = rotMatrix_Rear*velTire_RL;
velX_RL = vel_help_RL(1);
velY_RL = vel_help_RL(2);
vel_help_RR = rotMatrix_Rear*velTire_RR;
velX_RR = vel_help_RR(1);
velY_RR = vel_help_RR(2);

velX= single([velX_FL, velX_FR, velX_RL, velX_RR]);
velY= single([velY_FL, velY_FR, velY_RL, velY_RR]);



% relative velocities of wheels
velRelX_FL = WheelVelocity_FL - velX_FL;  %hier später die Zustände aus dem kalman filter für wheelspeeds
velRelX_FR = WheelVelocity_FR - velX_FR;
velRelX_RL = WheelVelocity_RL  - velX_RL;
velRelX_RR = WheelVelocity_RR  - velX_RR;


if(velX*ones(4,1) < 0.4) %TODO: Nachschauen, ob die Schwelle Probleme bereitet, oder ob diese höher oder tiefer gesetzt werden muss
    TireSlipLong = single([0, 0, 0, 0].');
end   
if(VelX< 0.4) %TODO: Nachschauen, ob die Schwelle Probleme bereitet, oder ob diese höher oder tiefer gesetzt werden muss
    TireSlipLong = single([0, 0, 0, 0].');
end 

for n=1:1:4
    if TireSlipLong(n) > 1
        TireSlipLong(n) = 1;
    elseif TireSlipLong(n) < -1
        TireSlipLong(n) = -1;
    end
end
end

== matlab function test_com_SensorFusion_SF_D4_ukf/Subsystem14/SensorFusion_D4/MATLAB Function1 ==
  data: u input; y output
function y = fcn(u)
a=5;
b=14;
y=filter(b, a, u);
end

== matlab function test_com_SensorFusion_SF_D4_ukf/Subsystem14/SensorFusion_D4/MATLAB Function2 ==
  data: WheelSpeeds input; WheelSpeeds_Sq input; WheelSpeeds_filtered output; dt input
function WheelSpeeds_filtered =  fc( WheelSpeeds, WheelSpeeds_Sq, dt)

persistent x P								

%Variablen für bias Messung
persistent standstill_counter
persistent bias_measurements 
persistent P_bias




%%
num_states=4;
num_measurements=4;
if isempty(P)
   
    
    
    %% bias Variablen Initialisierung
    P_bias=eye(num_measurements)*0.001;
    standstill_counter=0;
    bias_measurements=single(zeros(num_measurements,1));
    
    
    x = single(zeros(num_states,1));
    P = single(zeros(num_states, num_states));
	
  
end


%% Readability

    WheelVelocity_FL=x(1);
    WheelVelocity_FR=x(2);
    WheelVelocity_RL=x(3);
    WheelVelocity_RR=x(4);
    

    measurements= [
WheelSpeeds(1)      % (16)  wheelspeed  FL
WheelSpeeds(2)      % (17)  wheelspeed  FR
WheelSpeeds(3)      % (18)  wheelspeed  RL
WheelSpeeds(4)      % (19)  wheelspeed  RR
];

measurements_Sq= [
WheelSpeeds_Sq(1)      % (16)  wheelspeed  FL               Signal Quality
WheelSpeeds_Sq(2)      % (17)  wheelspeed  FR               Signal Quality
WheelSpeeds_Sq(3)      % (18)  wheelspeed  RL               Signal Quality
WheelSpeeds_Sq(4)      % (19)  wheelspeed  RR               Signal Quality
];


%Correction of the sensor inputs with the estimated biases
% nb == no bias
measurements_nb=    measurements-bias_measurements;
WheelSpeeds_nb=     single(zeros(4,1));

    

WheelSpeeds_nb(1)=      measurements_nb(1);
WheelSpeeds_nb(2)=      measurements_nb(2);
WheelSpeeds_nb(3)=      measurements_nb(3);
WheelSpeeds_nb(4)=      measurements_nb(4);


							  
									  																			 %% Preparing WheelSpeeds


% Durchschnittliche Radgeschwindigkeiten ermitteln
avgWheelVelocity = mean(WheelSpeeds);








%% Prediction 

if(avgWheelVelocity < 0.01 )
        vehicle_is_driving=false;
        standstill_counter=standstill_counter+1;
    else
        vehicle_is_driving=true;
        standstill_counter=0;
end


if ~vehicle_is_driving
    
    if standstill_counter*dt>0.5 && standstill_counter*dt<10
        
    kill_matrix_bias=zeros(num_measurements,num_measurements);
        for i=1:num_measurements
            if measurements_Sq(i)<4
                kill_matrix_bias(i,i)=1;
            end
        end
%         kill_matrix_bias=zeros(num_measurements,num_measurements);
        H_bias=kill_matrix_bias;
        R_bias=eye(num_measurements)*0.01;  % Sinnvolle Werte?
        I_bias=eye(num_measurements);
        
        Z_bias = kill_matrix_bias*measurements;
        w_bias = Z_bias-(H_bias*bias_measurements);
        K_bias = (P_bias*H_bias')/(H_bias*P_bias*H_bias.'+R_bias);  
        bias_measurements = bias_measurements+K_bias*w_bias;
        P_bias = (I_bias-K_bias*H_bias)*P_bias;
    end

    else % update the state only if the biases are currently not measured
        

   x=[  x(1);                                              % YawAcc;(18)  YawAcceleration of the Monocoque          
        x(2);                                              % wheelVelocity_FL;(19)  wheelspeed front left  wheel in rad         
        x(3);                                              %  wheelVelocity_FR;(20)  wheelspeed front right wheel in rad         
        x(4)];                                             % wheelVelocity_RL;(21)  wheelspeed rear  left  wheel in rad           ];                                              % wheelVelocity_RR;(22)  wheelspeed rear  right wheel in rad


    %Calculating a linearized A Matrix
          %PosX           VelX                AccX          PosY         VelY        AccY PosZ        VelZ          AccZ RollAngle  RollRate  RollAcc PitchAn PitchRate PitchAcc  YawAngle                                    YawRate YawAcc  19  20  21  22
    A=eye(4); 


    W = eye(num_states);

%     exp=single(0.4/((0.2*(x(5)-1)^2)+1)-2.4);%(0.4*(2^(-0.1*(x(5)-1)^2))-3.1);%-2.7*2^(-0.1*(x(5)-1)^2)-3.1*(-2^(-0.1*(x(5)-1)^2)+1) % This exponent is a value between -2.1 (if x(5)=2) and -4.5 (if x(5) is away from 2)
    % Covariance matrix of state noise
 Q = diag([
            1;       %WheelspeedFL;    % (19)  
            1;       %WheelspeedFR;    % (20)  
            1;       %WheedspeedRL;    % (21)  
            1]*0.001);  %WheelspeedRR;    % (22)   %dt
            

    % prediction calculation
    %x = x + dt*F*x; % + dt*B*u;          % statevector update
    %NO LINEAR EQUOTATION USED, THEREFORE ONLY THE LINEARIZED MATRIX A IS USED
    %TO UPDATE P

    P = A*P*A' + W*Q*W';                 % covariance matrix update
				   
end 


   

%% Measurement SF
% Measurement selection: With the help of the singal qualifiers it is
% determined which signal can be used as a measurement input for the kalman
% filter
%% Start der States
% Position X wird später bei uns von GPS gemessen noch kein info wie genau,
% bei Start wird Position auf null gesetzt
selection=[];

% WheelSpeeds (19) Front Left
if WheelSpeeds_Sq(1)<3
    WheelVelocity_FL_measurement=WheelSpeeds_nb(1);
    R_WheelVelocity_FL=0.0001;
    selection=[selection 1];
elseif WheelSpeeds_Sq(1)>4 && WheelSpeeds_Sq(2)<3 && WheelSpeeds_Sq(3)<3 && WheelSpeeds_nb(4)<3
    WheelVelocity_FL_measurement=(WheelSpeeds_nb(2)+WheelSpeeds_nb(3)+WheelSpeeds_nb(4))/3;%tire_r_dyn*
    R_WheelVelocity_FL=0.0001;
    selection=[selection 1];
else
    WheelVelocity_FL_measurement=single(0);
    R_WheelVelocity_FL=0.001;
end

% WheelSpeeds (20) Front Left
if WheelSpeeds_Sq(2)<3
    WheelVelocity_FR_measurement=WheelSpeeds_nb(2);
    R_WheelVelocity_FR=0.0001;
    selection=[selection 2];
elseif WheelSpeeds_Sq(2)>4 && WheelSpeeds_Sq(1)<3 && WheelSpeeds_Sq(3)<3 && WheelSpeeds_nb(4)<3
    WheelVelocity_FR_measurement= (WheelSpeeds_nb(1)+WheelSpeeds_nb(3)+WheelSpeeds_nb(4))/3;
    R_WheelVelocity_FR=0.0001;
    selection=[selection 2];
else
    WheelVelocity_FR_measurement=single(0);
    R_WheelVelocity_FR=0.1;
end

% WheelSpeeds (21) Front Left
if WheelSpeeds_Sq(3)<3
    WheelVelocity_RL_measurement=WheelSpeeds_nb(3);
    R_WheelVelocity_RL=0.0001;
    selection=[selection 3];
elseif WheelSpeeds_Sq(3)>4 && WheelSpeeds_Sq(1)<3 && WheelSpeeds_Sq(2)<3 && WheelSpeeds_nb(4)<3
    WheelVelocity_RL_measurement= (WheelSpeeds_nb(1)+WheelSpeeds_nb(2)+WheelSpeeds_nb(4))/3;
    R_WheelVelocity_RL=0.0001;
    selection=[selection 3];
else
    WheelVelocity_RL_measurement=single(0);
    R_WheelVelocity_RL=0.0001;
end
% WheelSpeeds (22) Front Left
if WheelSpeeds_Sq(4)<3
    WheelVelocity_RR_measurement=WheelSpeeds_nb(4);
    R_WheelVelocity_RR=0.0001;
    selection=[selection 4];
elseif WheelSpeeds_Sq(4)>4 && WheelSpeeds_Sq(1)<3 && WheelSpeeds_Sq(3)<3 && WheelSpeeds_nb(3)<3
    WheelVelocity_RR_measurement= (WheelSpeeds_nb(1)+WheelSpeeds_nb(3)+WheelSpeeds_nb(3))/3;
    R_WheelVelocity_RR=0.0001;
    selection=[selection 4];
else
  WheelVelocity_RR_measurement=single(0);
    R_WheelVelocity_RR=0.0001;
end



% Measured states
    
z1 = [ WheelVelocity_FL_measurement;     % WheelspeedFL (19)
      WheelVelocity_FR_measurement;     %WheelspeedFR  (20)
      WheelVelocity_RL_measurement;     %WheelspeedRL  (21)
      WheelVelocity_RR_measurement;   %WheelspeedRR (22)
    ];    
  

kill_matrix=zeros(length(z1),length(z1));
z=single(zeros(size(z1)));

for w=1:length(selection)
    z(selection(w))=z1(selection(w));    
    kill_matrix(selection(w),selection(w))=1.0;
end

h1=x;
h=kill_matrix*h1;

R = diag([
    1;                             % für die RH vgl mit RollANgle, PitchANgle und PosZ0.0
    1;
    1;
    1]);                    
H=eye(length(x));

% Correction equations
I = eye(length(x));
V = eye(length(z));

K_tmp = P*H'/(H*P*H'+V*R*V');

x = x + K_tmp*(z-h);
P = (I - K_tmp*H)*P;
WheelSpeeds_filtered=x;

== matlab function test_com_SensorFusion_SF_D4_ukf/Subsystem14/SensorFusion_D4/MATLAB Function3 ==
  data: AccX input; AccX_filtered output
function AccX_filtered = fcn(AccX)
persistent x P

if isempty(P)
    P=single(0);
end

Q=0.001;
A=1;

    W = eye(1);


    P = A*P*A' + W*Q*W';                 % covariance matrix update
				   
end 

% Measured states
    
z = AccX;    
  
h=x;
R = 1;                  
H=eye(length(x));

% Correction equations
I = eye(length(x));
V = eye(length(z));

K_tmp = P*H'/(H*P*H'+V*R*V');

x = x + K_tmp*(z-h);
P = (I - K_tmp*H)*P;

x=AccX_filtered;

== matlab function test_com_SensorFusion_SF_D4_ukf/Subsystem14/SensorFusion_D4/MATLAB Function4 ==
  data: AccX_Sq input; VD_diag_9Drear output; AccY_Sq input; AccZ_Sq input; YawRate_Sq input; PitchRate_Sq input; RollRate_Sq input
function VD_diag_9Drear = diag(AccX_Sq, AccY_Sq, AccZ_Sq, YawRate_Sq, PitchRate_Sq, RollRate_Sq)
bad_Sq_counter=single(0);
VD_diag_9Drear=0;
persistent timestep_counter_old
if isempty(timestep_counter_old)
    timestep_counter_old=0;
end


if AccX_Sq>4
    bad_Sq_counter=bad_Sq_counter+1;
end
if AccY_Sq>4
    bad_Sq_counter=bad_Sq_counter+1;
end
if AccZ_Sq>4
    bad_Sq_counter=bad_Sq_counter+1;
end
if YawRate_Sq>4
    bad_Sq_counter=bad_Sq_counter+1;
end
if RollRate_Sq>4
    bad_Sq_counter=bad_Sq_counter+1;
end
if PitchRate_Sq>4
    bad_Sq_counter=bad_Sq_counter+1;
end

if  bad_Sq_counter>3
    timestep_counter=timestep_counter_old+1;
else 
    timestep_counter=0;
end


if bad_Sq_counter>3 && timestep_counter >4
    VD_diag_9Drear=1;
end

timestep_counter_old=timestep_counter;

end

== matlab function test_com_SensorFusion_SF_D4_ukf/Subsystem14/SensorFusion_D4/MATLAB Function5 ==
  data: VelX_Sq input; VD_diag_v2o output; VelY_Sq input; bad_Sq_counter output; timestep_counter output
function [VD_diag_v2o, bad_Sq_counter, timestep_counter] = diag(VelX_Sq, VelY_Sq)
bad_Sq_counter=single(0);
VD_diag_v2o=0;
persistent timestep_counter_old
if isempty(timestep_counter_old)
    timestep_counter_old=0;
end

if VelX_Sq>4
    bad_Sq_counter=bad_Sq_counter+1;
end
if VelY_Sq>4
    bad_Sq_counter=bad_Sq_counter+1;
end

if  bad_Sq_counter>1
    timestep_counter=timestep_counter_old+1;
else 
    timestep_counter=0;
end

if bad_Sq_counter>1 && timestep_counter >4
    VD_diag_v2o=1;
end

timestep_counter_old=timestep_counter;

end

== matlab function test_com_SensorFusion_SF_D4_ukf/Subsystem14/SensorFusion_D4/MATLAB Function6 ==
  data: AccX_Sq input; VD_diag_9Dfront output; AccY_Sq input; AccZ_Sq input; YawRate_Sq input; PitchRate_Sq input; RollRate_Sq input
function VD_diag_9Dfront = diag(AccX_Sq, AccY_Sq, AccZ_Sq, YawRate_Sq, PitchRate_Sq, RollRate_Sq)
bad_Sq_counter=single(0);
VD_diag_9Dfront=0;
persistent timestep_counter_old
if isempty(timestep_counter_old)
    timestep_counter_old=0;
end


if AccX_Sq>4
    bad_Sq_counter=bad_Sq_counter+1;
end
if AccY_Sq>4
    bad_Sq_counter=bad_Sq_counter+1;
end
if AccZ_Sq>4
    bad_Sq_counter=bad_Sq_counter+1;
end
if YawRate_Sq>4
    bad_Sq_counter=bad_Sq_counter+1;
end
if RollRate_Sq>4
    bad_Sq_counter=bad_Sq_counter+1;
end
if PitchRate_Sq>4
    bad_Sq_counter=bad_Sq_counter+1;
end

if  bad_Sq_counter>3
    timestep_counter=timestep_counter_old+1;
else 
    timestep_counter=0;
end
if bad_Sq_counter>3 && timestep_counter >4
    VD_diag_9Dfront=1;
end

timestep_counter_old=timestep_counter;

end

== matlab function test_com_SensorFusion_SF_D4_ukf/Subsystem14/SensorFusion_D4/MATLAB Function7 ==
  data: RockerAngle_FL_Sq input; VD_diag_RockerAngle output; RockerAngle_FR_Sq input; bad_Sq_counter output; timestep_counter output; RockerAngle_RL_Sq input; RockerAngle_RR_Sq input
function [VD_diag_RockerAngle, bad_Sq_counter, timestep_counter] = diag(RockerAngle_FL_Sq, RockerAngle_FR_Sq, RockerAngle_RL_Sq, RockerAngle_RR_Sq)
bad_Sq_counter=single(0);
VD_diag_RockerAngle=0;
persistent timestep_counter_old
if isempty(timestep_counter_old)
    timestep_counter_old=0;
end

if RockerAngle_FL_Sq>4
    bad_Sq_counter=bad_Sq_counter+1;
end
if RockerAngle_FR_Sq>4
    bad_Sq_counter=bad_Sq_counter+1;
end
if RockerAngle_RL_Sq>4
    bad_Sq_counter=bad_Sq_counter+1;
end
if RockerAngle_RR_Sq>4
    bad_Sq_counter=bad_Sq_counter+1;
end

if  bad_Sq_counter>1
    timestep_counter=timestep_counter_old+1;
else 
    timestep_counter=0;
end

if bad_Sq_counter>1 && timestep_counter >4
    VD_diag_RockerAngle=1;
end

timestep_counter_old=timestep_counter;

end
